simulink model "meat_1024pt_bee2_fpv3"  (Simulink 6.2)
settings: Solver=ode45  StartTime=0.0  StopTime=60000  RelTol=1e-3
undefined symbols (not defined in the file): BEE2_usr, bit_rev, pfb_coeff_gen_calc
libraries: xbsIndex_r3 x1085, casper_library x94, xps_library x27
(part 3 of 8)

== system meat_1024pt_bee2_fpv3/vacc2 ==
  note: The slice selects the upper bits of the
      | counter which represent the vector number.
  note: Acc Len is the total number of vectors accumulated minus one
      | Thus acc_len = 0 causes no accumulation, the data is passed through
  note: Valid goes high when dout
      | represents a valid accumulation
  note: ValidDelay should be equal to
      | Add Latency + Mux Latency to align the valid pulse with the output data.
  note: We want to generate a sync pulse that
      | will reset the counter right when the low bits
      | would roll over from veclen-1 to 0 so we need
      | to compare to veclen-2 to take into account
      | the latency in the comparator
  sync : Inport  Port=1  LatchInput=off
  din : Inport  Port=2  LatchInput=off
  acc_len : Inport  Port=3  LatchInput=off
  AND : xbsIndex_r3/Logical  logical_function=AND  inputs=2  precision=Full  arith_type=Unsigned  n_bits=8  bin_pt=2  align_bp=on  latency=0  explicit_period=off  period=1  en=off  dbl_ovrd=off  show_param=off
      settings: xl_area=[0, 0, 0, 0, 0, 0, 0]
  AccEnCompare : xbsIndex_r3/Relational  mode=a!=b  latency=1  explicit_period=off  period=1  en=off  dbl_ovrd=off  show_param=off
      settings: xl_area=[0, 0, 0, 0, 0, 0, 0]
  Counter : xbsIndex_r3/Counter  cnt_type=Free Running  n_bits=20  bin_pt=0  arith_type=Unsigned  start_count=0  cnt_to=Inf  cnt_by_val=1  operation=Up  explicit_period=on  period=1  load_pin=off  rst=on  en=off  dbl_ovrd=off  show_param=off  use_rpm=on  gen_core=off
      settings: xl_area=[0, 0, 0, 0, 0, 0, 0]
  Cram : Subsystem  AncestorBlock=gavrt_library/cram  mask(cram){num_slice=2}
      mask prompts: num_slice "Number of slices"
      mask help: Concatenates inputs together after forcing binary point to zero.
      mask init:
      | cram_init(gcb, ...
      |     'num_slice', num_slice);
  DinDelay : xbsIndex_r3/Delay  latency=2  reg_retiming=on  explicit_period=off  period=1  en=off  accept_only_valid=off  init_zero=on  dbl_ovrd=off  show_param=off
      settings: xl_area=[0, 0, 0, 0, 0, 0, 0]
  OR : xbsIndex_r3/Logical  logical_function=OR  inputs=2  precision=Full  arith_type=Unsigned  n_bits=8  bin_pt=2  align_bp=on  latency=0  explicit_period=off  period=1  en=off  dbl_ovrd=off  show_param=off
      settings: xl_area=[0, 0, 0, 0, 0, 0, 0]
  Slice : xbsIndex_r3/Slice  mode=Upper Bit Location + Width  nbits=10  bit1=0  base1=MSB of Input  bit0=0  base0=LSB of Input  boolean_output=off  explicit_period=off  period=1  dbl_ovrd=off
  SliceLow : xbsIndex_r3/Slice  mode=Lower Bit Location + Width  nbits=10  bit1=0  base1=MSB of Input  bit0=0  base0=LSB of Input  boolean_output=off  explicit_period=off  period=1  dbl_ovrd=off
  SyncCompare : xbsIndex_r3/Relational  mode=a=b  latency=1  explicit_period=off  period=1  en=off  dbl_ovrd=off  show_param=off
      settings: xl_area=[0, 0, 0, 0, 0, 0, 0]
  SyncConst : xbsIndex_r3/Constant  const=1022  equ=P=C  arith_type=Unsigned  n_bits=10  bin_pt=0  opselect=C  inp2=PCIN>>17  opr=+  inp1=P  carry=CIN  iostate=0  explicit_period=on  period=1  dbl_ovrd=off
  SyncDelay : xbsIndex_r3/Delay  latency=0  reg_retiming=off  explicit_period=off  period=1  en=off  accept_only_valid=off  init_zero=on  dbl_ovrd=off  show_param=off
      settings: xl_area=[0, 0, 0, 0, 0, 0, 0]
  Uncram : Subsystem  AncestorBlock=gavrt_library/uncram  mask(uncram){num_slice=2, slice_width=48, bin_pt=46, arith_type=0}
      mask prompts: num_slice "Number of slices"; slice_width "Slice Width"; bin_pt "Output Binary Point"; arith_type "Output Arithmetic Type (0=Unsigned, 1=Signed, 2=Boolean)"
      mask help: Takes a concatenated input and slices it up into even pieces and reinterprets them as signed fixed point numbers with a given binary point.
      mask init:
      | uncram_init(gcb, ...
      |     'num_slice', num_slice, ...
      |     'slice_width', slice_width, ...
      |     'bin_pt', bin_pt, ...
      |     'arith_type', arith_type);
      settings: AttributesFormatString=UFix_48_46
  ValidCompare : xbsIndex_r3/Relational  mode=a=b  latency=1  explicit_period=off  period=1  en=off  dbl_ovrd=off  show_param=off
      settings: xl_area=[0, 0, 0, 0, 0, 0, 0]
  ValidDelay : xbsIndex_r3/Delay  latency=3  reg_retiming=off  explicit_period=off  period=1  en=off  accept_only_valid=off  init_zero=on  dbl_ovrd=off  show_param=off
      settings: xl_area=[0, 0, 0, 0, 0, 0, 0]
  Zero : xbsIndex_r3/Constant  const=0  equ=P=C  arith_type=Unsigned  n_bits=8  bin_pt=0  opselect=C  inp2=PCIN>>17  opr=+  inp1=P  carry=CIN  iostate=0  explicit_period=on  period=1  dbl_ovrd=off
  vacc_core1 : Subsystem  AncestorBlock=gavrt_library/vacc_core  mask(vacc_core){veclen=1024, arith_type=0, out_bit_width=64, out_bin_pt=46, add_latency=2, bram_latency=2, mux_latency=1}
      mask prompts: veclen "Vector Length"; arith_type "Arithmetic Type (0=Unsigned, 1=Signed)"; out_bit_width "Output Bit Width"; out_bin_pt "Output Binary Point"; add_latency "Add Latency"; bram_latency "BRAM Latency"; mux_latency "Mux Latency"
      mask help:
      | Currently only Signed arithmetic supported
      | acc_en = 0 --> Load a vector (start a new accumulation)
      | acc_en = 1 --> Accumulate
      mask init: same as meat_1024pt_bee2_fpv3/vacc/vacc_core1
  vacc_core2 : Subsystem  AncestorBlock=gavrt_library/vacc_core  mask(vacc_core){veclen=1024, arith_type=0, out_bit_width=64, out_bin_pt=46, add_latency=2, bram_latency=2, mux_latency=1}
      mask prompts: veclen "Vector Length"; arith_type "Arithmetic Type (0=Unsigned, 1=Signed)"; out_bit_width "Output Bit Width"; out_bin_pt "Output Binary Point"; add_latency "Add Latency"; bram_latency "BRAM Latency"; mux_latency "Mux Latency"
      mask help:
      | Currently only Signed arithmetic supported
      | acc_en = 0 --> Load a vector (start a new accumulation)
      | acc_en = 1 --> Accumulate
      mask init: same as meat_1024pt_bee2_fpv3/vacc/vacc_core1
  valid : Outport
  dout : Outport  Port=2
  wires:
  sync/1 -> SyncDelay/1
  SyncDelay/1 -> OR/1
  [valid] -> AND/1
  AND/1 -> OR/2
  OR/1 -> Counter/1
  Counter/1 -> [count], Slice/1
  [count] -> SliceLow/1
  SliceLow/1 -> SyncCompare/1
  SyncConst/1 -> SyncCompare/2
  SyncCompare/1 -> AND/2
  ValidCompare/1 -> [valid], ValidDelay/1
  acc_len/1 -> ValidCompare/1
  Slice/1 -> ValidCompare/2, AccEnCompare/1
  Zero/1 -> AccEnCompare/2
  ValidDelay/1 -> valid/1
  din/1 -> DinDelay/1
  DinDelay/1 -> Uncram/1(In)
  Cram/1(Out) -> dout/1
  Uncram/1(Out1) -> vacc_core1/1(din)
  AccEnCompare/1 -> vacc_core1/2(acc_en), vacc_core2/2(acc_en)
  vacc_core1/1(dout) -> Cram/1(In1)
  Uncram/2(Out2) -> vacc_core2/1(din)
  vacc_core2/1(dout) -> Cram/2(In2)

== system meat_1024pt_bee2_fpv3/StokesDetector/XMultiply_f0 ==
  Pol1 : Inport  Port=1  LatchInput=off
  Pol2 : Inport  Port=2  LatchInput=off
  add : xbsIndex_r3/AddSub  mode=Addition  precision=User Defined  arith_type="Signed  (2's comp)"  n_bits=32  bin_pt=31  quantization="Round  (unbiased: +/- Inf)"  overflow=Wrap  latency=2  explicit_period=off  period=1  use_carryin=off  use_carryout=off  en=off  dbl_ovrd=off  show_param=off  use_core=on  pipeline=off  use_rpm=on  gen_core=off
      settings: xl_area=[0, 0, 0, 0, 0, 0, 0]
  c_to_ri : casper_library/Misc/c_to_ri  n_bits=18  bin_pt=17
      settings: AttributesFormatString=18_17 r/i
  c_to_ri1 : casper_library/Misc/c_to_ri  n_bits=18  bin_pt=17
      settings: AttributesFormatString=18_17 r/i
  mult{1..4} (4 alike) : xbsIndex_r3/Mult  precision=Full  arith_type="Signed  (2's comp)"  n_bits=8  bin_pt=2  quantization=Truncate  overflow=Wrap  latency=3  explicit_period=off  period=1  en=off  dbl_ovrd=off  show_param=on  mult_type=Parallel  oversample=2  use_embedded=on  pipeline=on  use_rpm=on  placement_style=Rectangular Shape  gen_core=off
      settings: xl_area=[0, 0, 0, 0, 0, 0, 0]
  sub : xbsIndex_r3/AddSub  mode=Subtraction  precision=User Defined  arith_type="Signed  (2's comp)"  n_bits=32  bin_pt=31  quantization="Round  (unbiased: +/- Inf)"  overflow=Wrap  latency=2  explicit_period=off  period=1  use_carryin=off  use_carryout=off  en=off  dbl_ovrd=off  show_param=off  use_core=on  pipeline=off  use_rpm=on  gen_core=off
      settings: xl_area=[0, 0, 0, 0, 0, 0, 0]
  X Real : Outport
  X Imag : Outport  Port=2
  wires:
  c_to_ri/1 -> mult1/1, mult2/1
  c_to_ri1/1 -> mult1/2, mult3/2
  c_to_ri/2 -> mult3/1, mult4/1
  c_to_ri1/2 -> mult2/2, mult4/2
  mult4/1 -> add/1
  mult1/1 -> add/2
  mult2/1 -> sub/1
  mult3/1 -> sub/2
  Pol1/1 -> c_to_ri/1
  Pol2/1 -> c_to_ri1/1
  add/1 -> X Real/1
  sub/1 -> X Imag/1

== system meat_1024pt_bee2_fpv3/StokesDetector/pol1_power0 ==
  note: Power - Unsigned Output
  c : Inport  Port=1  LatchInput=off
  c_to_ri : casper_library/Misc/c_to_ri  n_bits=18  bin_pt=17
      settings: AttributesFormatString=18_17 r/i
  imag_square : xbsIndex_r3/Mult  precision=Full  arith_type="Signed  (2's comp)"  n_bits=18  bin_pt=17  quantization=Truncate  overflow=Wrap  latency=3  explicit_period=off  period=1  en=off  dbl_ovrd=off  show_param=on  mult_type=Parallel  oversample=2  use_embedded=on  pipeline=on  use_rpm=on  placement_style=Rectangular Shape  gen_core=off
      settings: xl_area=[0, 0, 0, 0, 0, 0, 0]
  power_adder : xbsIndex_r3/AddSub  mode=Addition  precision=User Defined  arith_type=Unsigned  n_bits=32  bin_pt=31  quantization="Round  (unbiased: +/- Inf)"  overflow=Wrap  latency=2  explicit_period=off  period=1  use_carryin=off  use_carryout=off  en=off  dbl_ovrd=off  show_param=off  use_core=on  pipeline=off  use_rpm=on  gen_core=off
      settings: xl_area=[0, 0, 0, 0, 0, 0, 0]
  real_square : xbsIndex_r3/Mult  precision=Full  arith_type="Signed  (2's comp)"  n_bits=18  bin_pt=17  quantization=Truncate  overflow=Wrap  latency=3  explicit_period=off  period=1  en=off  dbl_ovrd=off  show_param=on  mult_type=Parallel  oversample=2  use_embedded=on  pipeline=on  use_rpm=on  placement_style=Rectangular Shape  gen_core=off
      settings: xl_area=[0, 0, 0, 0, 0, 0, 0]
  power : Outport
  wires:
  imag_square/1 -> power_adder/2
  real_square/1 -> power_adder/1
  c_to_ri/1 -> real_square/1, real_square/2
  c_to_ri/2 -> imag_square/2, imag_square/1
  c/1 -> c_to_ri/1
  power_adder/1 -> power/1

== system meat_1024pt_bee2_fpv3/StokesDetector/pol2_power0 ==
  note: Power - Unsigned Output
  c : Inport  Port=1  LatchInput=off
  c_to_ri : casper_library/Misc/c_to_ri  n_bits=18  bin_pt=17
      settings: AttributesFormatString=18_17 r/i
  imag_square : xbsIndex_r3/Mult  precision=Full  arith_type="Signed  (2's comp)"  n_bits=18  bin_pt=17  quantization=Truncate  overflow=Wrap  latency=3  explicit_period=off  period=1  en=off  dbl_ovrd=off  show_param=on  mult_type=Parallel  oversample=2  use_embedded=on  pipeline=on  use_rpm=on  placement_style=Rectangular Shape  gen_core=off
      settings: xl_area=[0, 0, 0, 0, 0, 0, 0]
  power_adder : xbsIndex_r3/AddSub  mode=Addition  precision=User Defined  arith_type=Unsigned  n_bits=32  bin_pt=31  quantization="Round  (unbiased: +/- Inf)"  overflow=Wrap  latency=2  explicit_period=off  period=1  use_carryin=off  use_carryout=off  en=off  dbl_ovrd=off  show_param=off  use_core=on  pipeline=off  use_rpm=on  gen_core=off
      settings: xl_area=[0, 0, 0, 0, 0, 0, 0]
  real_square : xbsIndex_r3/Mult  precision=Full  arith_type="Signed  (2's comp)"  n_bits=18  bin_pt=17  quantization=Truncate  overflow=Wrap  latency=3  explicit_period=off  period=1  en=off  dbl_ovrd=off  show_param=on  mult_type=Parallel  oversample=2  use_embedded=on  pipeline=on  use_rpm=on  placement_style=Rectangular Shape  gen_core=off
      settings: xl_area=[0, 0, 0, 0, 0, 0, 0]
  power : Outport
  wires:
  power_adder/1 -> power/1
  c/1 -> c_to_ri/1
  c_to_ri/2 -> imag_square/1, imag_square/2
  c_to_ri/1 -> real_square/2, real_square/1
  real_square/1 -> power_adder/1
  imag_square/1 -> power_adder/2

== system meat_1024pt_bee2_fpv3/fft/fft_biplex0 ==
  pol1 : Inport  Port=1  LatchInput=off
  pol2 : Inport  Port=2  LatchInput=off
  sync : Inport  Port=3  LatchInput=off
  shift : Inport  Port=4  LatchInput=off
  biplex_core : Subsystem  AncestorBlock=casper_library/FFTs/biplex_core  mask(biplex_core){FFTSize=10, BitWidth=18, quantization=Truncate, overflow=Wrap, add_latency=3, mult_latency=4, bram_latency=3}
      mask prompts: FFTSize "Size of FFT: (2^? pnts)"; BitWidth "Bitwidth: (Max Efficiency at 18 bits)"; quantization "Quantization Behavior"; overflow "Overflow Behavior"; add_latency "Add Latency"; mult_latency "Mult Latency"; bram_latency "BRAM Latency"
      mask init:
      | biplex_core_init(gcb,...
      |     'FFTSize', FFTSize,...
      |     'BitWidth', BitWidth,...
      |     'quantization', quantization,...
      |     'overflow', overflow,...
      |     'add_latency', add_latency,...
      |     'mult_latency', mult_latency,...
      |     'bram_latency', bram_latency);
      settings: AttributesFormatString=FFTSize=10
      mask StyleString: edit,edit,popup(Truncate|Round  (unbiased: +/- Inf)|Round  (unbiased: Even Values)),popup(Wrap|Saturate|Error),edit,edit,edit
  biplex_cplx_unscrambler : Subsystem  mask{FFTSize=10, bram_latency=3}
      mask prompts: FFTSize "Size of FFT: (2^? pnts)"; bram_latency "BRAM Latency"
      mask init:
      | blk = gcb;
      | map = bit_reverse(0:2^(FFTSize-1)-1, FFTSize-1);
      | set_param([blk,'/reorder'],'map',mat2str([map,map+2^(FFTSize-1)]));
      | set_param([blk,'/reorder'],'bram_latency', num2str(bram_latency));
      | set_param([blk,'/reorder1'],'map',mat2str([map+2^(FFTSize-1),map]));
      | set_param([blk,'/reorder1'],'bram_latency', num2str(bram_latency));
  pol1_out : Outport
  pol2_out : Outport  Port=2
  of : Outport  Port=3
  sync_out : Outport  Port=4
  wires:
  biplex_cplx_unscrambler/3(sync_out) -> sync_out/1
  biplex_cplx_unscrambler/2(pol2) -> pol2_out/1
  biplex_core/4(sync_out) -> biplex_cplx_unscrambler/3(sync)
  biplex_core/2(out2) -> biplex_cplx_unscrambler/2(odd)
  biplex_core/1(out1) -> biplex_cplx_unscrambler/1(even)
  pol1/1 -> biplex_core/1(pol1)
  pol2/1 -> biplex_core/2(pol2)
  sync/1 -> biplex_core/3(sync)
  shift/1 -> biplex_core/4(shift)
  biplex_cplx_unscrambler/1(pol1) -> pol1_out/1
  biplex_core/3(of) -> of/1

== system meat_1024pt_bee2_fpv3/pfb_fir/pol1_in1_first_tap ==
  din : Inport  Port=1  LatchInput=off
  sync : Inport  Port=2  LatchInput=off
  Mult : xbsIndex_r3/Mult  precision=Full  arith_type="Signed  (2's comp)"  n_bits=8  bin_pt=2  quantization=Truncate  overflow=Wrap  latency=mult_latency  explicit_period=off  period=1  en=off  dbl_ovrd=off  show_param=on  mult_type=Parallel  oversample=2  use_embedded=on  pipeline=on  use_rpm=on  placement_style=Rectangular Shape  gen_core=off
      settings: xl_area=[0, 0, 0, 0, 0, 0, 0]
  Mult1 : xbsIndex_r3/Mult  precision=Full  arith_type="Signed  (2's comp)"  n_bits=8  bin_pt=2  quantization=Truncate  overflow=Wrap  latency=mult_latency  explicit_period=off  period=1  en=off  dbl_ovrd=off  show_param=on  mult_type=Parallel  oversample=2  use_embedded=on  pipeline=on  use_rpm=on  placement_style=Rectangular Shape  gen_core=off
      settings: xl_area=[0, 0, 0, 0, 0, 0, 0]
  Reinterpret : xbsIndex_r3/Reinterpret  force_arith_type=on  arith_type="Signed  (2's comp)"  force_bin_pt=on  bin_pt=CoeffBitWidth - 1  force_valid=on
  Slice : xbsIndex_r3/Slice  mode=Lower Bit Location + Width  nbits=CoeffBitWidth  bit1=0  base1=MSB of Input  bit0=0  base0=LSB of Input  boolean_output=off  explicit_period=off  period=1  dbl_ovrd=off
  Slice1 : xbsIndex_r3/Slice  mode=Two Bit Locations  nbits=CoeffBitWidth * (TotalTaps - 1)  bit1=0  base1=MSB of Input  bit0=CoeffBitWidth  base0=LSB of Input  boolean_output=off  explicit_period=off  period=1  dbl_ovrd=off
  c_to_ri : casper_library/Misc/c_to_ri  n_bits=BitWidthIn  bin_pt=BitWidthIn-1
      settings: AttributesFormatString=8_7 r/i
  delay : Subsystem  BlockChoice=delay_bram
      link override delay_bram: DelayLen=2^(PFBSize-n_inputs)  bram_latency=bram_latency
      link override delay_bram/Constant2: equ=P=C
      settings: AttributesFormatString=%<BlockChoice>  TemplateBlock=casper_library/Delays/delay  MemberBlocks=delay_bram,delay_slr
  pfb_coeff_gen : Subsystem  AncestorBlock=casper_library/PFBs/pfb_coeff_gen  mask(pfb_coeff_gen){PFBSize=10, CoeffBitWidth=8, TotalTaps=4, CoeffDistMem=1, WindowType=hamming, bram_latency=3, n_inputs=0, nput=0, fwidth=1}
      mask prompts: PFBSize "Size of PFB: (2^? pnts)"; CoeffBitWidth "Bitwidth of Coefficients:"; TotalTaps "Total Number of Taps:"; CoeffDistMem "Implement Coeff Gen in Distributed Memory"; WindowType "Windowing Function:"; bram_latency "BRAM Latency"; n_inputs "Number of Simultaneous Inputs: (2^?)"; nput "This is input number:"; fwidth "Bin Width (normal=1)"
      mask init:
      | pfb_coeff_gen_init(gcb, ...
      |     'PFBSize', PFBSize, ...
      |     'CoeffBitWidth', CoeffBitWidth, ...
      |     'TotalTaps', TotalTaps, ...
      |     'CoeffDistMem', CoeffDistMem, ...
      |     'WindowType', WindowType, ...
      |     'bram_latency', bram_latency, ...
      |     'n_inputs', n_inputs, ...
      |     'nput', nput, ...
      |     'fwidth', fwidth);
      settings: AttributesFormatString=PFBSize=10, n_inputs=0, taps=4
  ri_to_c : Subsystem
  sync_delay : casper_library/Delays/sync_delay  DelayLen=2^(PFBSize-n_inputs)
      link override Constant: equ=P=C
      link override Constant1: equ=P=C
      link override Constant2: equ=P=C
      link override Constant3: equ=P=C
  dout : Outport
  sync_out : Outport  Port=2
  coeff_out : Outport  Port=3
  taps_out : Outport  Port=4
  wires:
  ri_to_c/1(c) -> taps_out/1
  Mult/1 -> ri_to_c/2(im)
  Mult1/1 -> ri_to_c/1(re)
  c_to_ri/2 -> Mult/1
  c_to_ri/1 -> Mult1/1
  pfb_coeff_gen/3(coeff) -> Slice1/1, Slice/1
  pfb_coeff_gen/2(sync_out) -> sync_delay/1
  sync/1 -> pfb_coeff_gen/2(sync)
  pfb_coeff_gen/1(dout) -> delay/1(In1), c_to_ri/1
  din/1 -> pfb_coeff_gen/1(din)
  delay/1(Out1) -> dout/1
  sync_delay/1 -> sync_out/1
  Slice1/1 -> coeff_out/1
  Slice/1 -> Reinterpret/1
  Reinterpret/1 -> Mult1/2, Mult/2

== system meat_1024pt_bee2_fpv3/pfb_fir/pol1_in1_last_tap ==
  din : Inport  Port=1  LatchInput=off
  sync : Inport  Port=2  LatchInput=off
  coeff : Inport  Port=3  LatchInput=off
  taps : Inport  Port=4  LatchInput=off
  Concat : xbsIndex_r3/Concat  num_inputs=2  explicit_period=off  period=1  dbl_ovrd=off
  Delay : xbsIndex_r3/Delay  latency=mult_latency  reg_retiming=off  explicit_period=off  period=1  en=off  accept_only_valid=off  init_zero=on  dbl_ovrd=off  show_param=off
      settings: xl_area=[0, 0, 0, 0, 0, 0, 0]
  Mult : xbsIndex_r3/Mult  precision=Full  arith_type="Signed  (2's comp)"  n_bits=8  bin_pt=2  quantization=Truncate  overflow=Wrap  latency=mult_latency  explicit_period=off  period=1  en=off  dbl_ovrd=off  show_param=on  mult_type=Parallel  oversample=2  use_embedded=on  pipeline=on  use_rpm=on  placement_style=Rectangular Shape  gen_core=off
      settings: xl_area=[0, 0, 0, 0, 0, 0, 0]
  Mult1 : xbsIndex_r3/Mult  precision=Full  arith_type="Signed  (2's comp)"  n_bits=8  bin_pt=2  quantization=Truncate  overflow=Wrap  latency=mult_latency  explicit_period=off  period=1  en=off  dbl_ovrd=off  show_param=on  mult_type=Parallel  oversample=2  use_embedded=on  pipeline=on  use_rpm=on  placement_style=Rectangular Shape  gen_core=off
      settings: xl_area=[0, 0, 0, 0, 0, 0, 0]
  Reinterpret : xbsIndex_r3/Reinterpret  force_arith_type=on  arith_type="Signed  (2's comp)"  force_bin_pt=on  bin_pt=CoeffBitWidth - 1  force_valid=on
  c_to_ri : casper_library/Misc/c_to_ri  n_bits=BitWidthIn  bin_pt=BitWidthIn-1
      settings: AttributesFormatString=8_7 r/i
  pfb_add_tree : Subsystem  mask(pfb_add_tree){TotalTaps=4, BitWidthIn=8, BitWidthOut=18, CoeffBitWidth=8, add_latency=2, quantization=Truncate}
      mask prompts: TotalTaps "Total Number of Taps:"; BitWidthIn "Input Bitwidth:"; BitWidthOut "Output Bitwidth:"; CoeffBitWidth "Coeff Bitwidth:"; add_latency "Add Latency"; quantization "Quantization Behavior"
      mask init:
      | pfb_add_tree_init(gcb, ...
      |     'TotalTaps', TotalTaps, ...
      |     'BitWidthIn', BitWidthIn, ...
      |     'BitWidthOut', BitWidthOut, ...
      |     'CoeffBitWidth', CoeffBitWidth, ...
      |     'add_latency', add_latency, ...
      |     'quantization', quantization);
      settings: AttributesFormatString=taps=4, add_latency=2
  ri_to_c : Subsystem
  dout : Outport
  sync_out : Outport  Port=2
  wires:
  Reinterpret/1 -> Mult/2, Mult1/2
  coeff/1 -> Reinterpret/1
  Concat/1 -> pfb_add_tree/1(din)
  taps/1 -> Concat/2
  sync/1 -> Delay/1
  pfb_add_tree/1(dout) -> dout/1
  pfb_add_tree/2(sync_out) -> sync_out/1
  Delay/1 -> pfb_add_tree/2(sync)
  c_to_ri/1 -> Mult1/1
  c_to_ri/2 -> Mult/1
  din/1 -> c_to_ri/1
  Mult1/1 -> ri_to_c/1(re)
  Mult/1 -> ri_to_c/2(im)
  ri_to_c/1(c) -> Concat/1

== system meat_1024pt_bee2_fpv3/pfb_fir/pol2_in1_first_tap ==
  din : Inport  Port=1  LatchInput=off
  sync : Inport  Port=2  LatchInput=off
  Mult : xbsIndex_r3/Mult  precision=Full  arith_type="Signed  (2's comp)"  n_bits=8  bin_pt=2  quantization=Truncate  overflow=Wrap  latency=mult_latency  explicit_period=off  period=1  en=off  dbl_ovrd=off  show_param=on  mult_type=Parallel  oversample=2  use_embedded=on  pipeline=on  use_rpm=on  placement_style=Rectangular Shape  gen_core=off
      settings: xl_area=[0, 0, 0, 0, 0, 0, 0]
  Mult1 : xbsIndex_r3/Mult  precision=Full  arith_type="Signed  (2's comp)"  n_bits=8  bin_pt=2  quantization=Truncate  overflow=Wrap  latency=mult_latency  explicit_period=off  period=1  en=off  dbl_ovrd=off  show_param=on  mult_type=Parallel  oversample=2  use_embedded=on  pipeline=on  use_rpm=on  placement_style=Rectangular Shape  gen_core=off
      settings: xl_area=[0, 0, 0, 0, 0, 0, 0]
  Reinterpret : xbsIndex_r3/Reinterpret  force_arith_type=on  arith_type="Signed  (2's comp)"  force_bin_pt=on  bin_pt=CoeffBitWidth - 1  force_valid=on
  Slice : xbsIndex_r3/Slice  mode=Lower Bit Location + Width  nbits=CoeffBitWidth  bit1=0  base1=MSB of Input  bit0=0  base0=LSB of Input  boolean_output=off  explicit_period=off  period=1  dbl_ovrd=off
  Slice1 : xbsIndex_r3/Slice  mode=Two Bit Locations  nbits=CoeffBitWidth * (TotalTaps - 1)  bit1=0  base1=MSB of Input  bit0=CoeffBitWidth  base0=LSB of Input  boolean_output=off  explicit_period=off  period=1  dbl_ovrd=off
  c_to_ri : casper_library/Misc/c_to_ri  n_bits=BitWidthIn  bin_pt=BitWidthIn-1
      settings: AttributesFormatString=8_7 r/i
  delay : Subsystem  BlockChoice=delay_bram
      link override delay_bram: DelayLen=2^(PFBSize-n_inputs)  bram_latency=bram_latency
      link override delay_bram/Constant2: equ=P=C
      settings: AttributesFormatString=%<BlockChoice>  TemplateBlock=casper_library/Delays/delay  MemberBlocks=delay_bram,delay_slr
  pfb_coeff_gen : Subsystem  AncestorBlock=casper_library/PFBs/pfb_coeff_gen  mask(pfb_coeff_gen){PFBSize=10, CoeffBitWidth=8, TotalTaps=4, CoeffDistMem=1, WindowType=hamming, bram_latency=3, n_inputs=0, nput=0, fwidth=1}
      mask prompts: PFBSize "Size of PFB: (2^? pnts)"; CoeffBitWidth "Bitwidth of Coefficients:"; TotalTaps "Total Number of Taps:"; CoeffDistMem "Implement Coeff Gen in Distributed Memory"; WindowType "Windowing Function:"; bram_latency "BRAM Latency"; n_inputs "Number of Simultaneous Inputs: (2^?)"; nput "This is input number:"; fwidth "Bin Width (normal=1)"
      mask init: same as meat_1024pt_bee2_fpv3/pfb_fir/pol1_in1_first_tap/pfb_coeff_gen
      settings: AttributesFormatString=PFBSize=10, n_inputs=0, taps=4
  ri_to_c : Subsystem
  sync_delay : casper_library/Delays/sync_delay  DelayLen=2^(PFBSize-n_inputs)
      link override Constant: equ=P=C
      link override Constant1: equ=P=C
      link override Constant2: equ=P=C
      link override Constant3: equ=P=C
  dout : Outport
  sync_out : Outport  Port=2
  coeff_out : Outport  Port=3
  taps_out : Outport  Port=4
  wires:
  ri_to_c/1(c) -> taps_out/1
  Mult/1 -> ri_to_c/2(im)
  Mult1/1 -> ri_to_c/1(re)
  c_to_ri/2 -> Mult/1
  c_to_ri/1 -> Mult1/1
  pfb_coeff_gen/3(coeff) -> Slice1/1, Slice/1
  pfb_coeff_gen/2(sync_out) -> sync_delay/1
  sync/1 -> pfb_coeff_gen/2(sync)
  pfb_coeff_gen/1(dout) -> delay/1(In1), c_to_ri/1
  din/1 -> pfb_coeff_gen/1(din)
  delay/1(Out1) -> dout/1
  sync_delay/1 -> sync_out/1
  Slice1/1 -> coeff_out/1
  Slice/1 -> Reinterpret/1
  Reinterpret/1 -> Mult1/2, Mult/2

== system meat_1024pt_bee2_fpv3/pfb_fir/pol2_in1_last_tap ==
  din : Inport  Port=1  LatchInput=off
  sync : Inport  Port=2  LatchInput=off
  coeff : Inport  Port=3  LatchInput=off
  taps : Inport  Port=4  LatchInput=off
  Concat : xbsIndex_r3/Concat  num_inputs=2  explicit_period=off  period=1  dbl_ovrd=off
  Delay : xbsIndex_r3/Delay  latency=mult_latency  reg_retiming=off  explicit_period=off  period=1  en=off  accept_only_valid=off  init_zero=on  dbl_ovrd=off  show_param=off
      settings: xl_area=[0, 0, 0, 0, 0, 0, 0]
  Mult : xbsIndex_r3/Mult  precision=Full  arith_type="Signed  (2's comp)"  n_bits=8  bin_pt=2  quantization=Truncate  overflow=Wrap  latency=mult_latency  explicit_period=off  period=1  en=off  dbl_ovrd=off  show_param=on  mult_type=Parallel  oversample=2  use_embedded=on  pipeline=on  use_rpm=on  placement_style=Rectangular Shape  gen_core=off
      settings: xl_area=[0, 0, 0, 0, 0, 0, 0]
  Mult1 : xbsIndex_r3/Mult  precision=Full  arith_type="Signed  (2's comp)"  n_bits=8  bin_pt=2  quantization=Truncate  overflow=Wrap  latency=mult_latency  explicit_period=off  period=1  en=off  dbl_ovrd=off  show_param=on  mult_type=Parallel  oversample=2  use_embedded=on  pipeline=on  use_rpm=on  placement_style=Rectangular Shape  gen_core=off
      settings: xl_area=[0, 0, 0, 0, 0, 0, 0]
  Reinterpret : xbsIndex_r3/Reinterpret  force_arith_type=on  arith_type="Signed  (2's comp)"  force_bin_pt=on  bin_pt=CoeffBitWidth - 1  force_valid=on
  c_to_ri : casper_library/Misc/c_to_ri  n_bits=BitWidthIn  bin_pt=BitWidthIn-1
      settings: AttributesFormatString=8_7 r/i
  pfb_add_tree : Subsystem  mask(pfb_add_tree){TotalTaps=4, BitWidthIn=8, BitWidthOut=18, CoeffBitWidth=8, add_latency=2, quantization=Truncate}
      mask prompts: TotalTaps "Total Number of Taps:"; BitWidthIn "Input Bitwidth:"; BitWidthOut "Output Bitwidth:"; CoeffBitWidth "Coeff Bitwidth:"; add_latency "Add Latency"; quantization "Quantization Behavior"
      mask init: same as meat_1024pt_bee2_fpv3/pfb_fir/pol1_in1_last_tap/pfb_add_tree
      settings: AttributesFormatString=taps=4, add_latency=2
  ri_to_c : Subsystem
  dout : Outport
  sync_out : Outport  Port=2
  wires:
  Reinterpret/1 -> Mult/2, Mult1/2
  coeff/1 -> Reinterpret/1
  Concat/1 -> pfb_add_tree/1(din)
  taps/1 -> Concat/2
  sync/1 -> Delay/1
  pfb_add_tree/1(dout) -> dout/1
  pfb_add_tree/2(sync_out) -> sync_out/1
  Delay/1 -> pfb_add_tree/2(sync)
  c_to_ri/1 -> Mult1/1
  c_to_ri/2 -> Mult/1
  din/1 -> c_to_ri/1
  Mult1/1 -> ri_to_c/1(re)
  Mult/1 -> ri_to_c/2(im)
  ri_to_c/1(c) -> Concat/1

== system meat_1024pt_bee2_fpv3/vacc/Cram ==
  In1 : Inport  Port=1  LatchInput=off
  In2 : Inport  Port=2  LatchInput=off
  Concat : xbsIndex_r3/Concat  num_inputs=2  explicit_period=off  period=1  dbl_ovrd=off
  Reinterp1 : xbsIndex_r3/Reinterpret  force_arith_type=on  arith_type=Unsigned  force_bin_pt=on  bin_pt=0  force_valid=on
  Reinterp2 : xbsIndex_r3/Reinterpret  force_arith_type=on  arith_type=Unsigned  force_bin_pt=on  bin_pt=0  force_valid=on
  Out : Outport
  wires:
  Concat/1 -> Out/1
  In1/1 -> Reinterp1/1
  Reinterp1/1 -> Concat/1
  In2/1 -> Reinterp2/1
  Reinterp2/1 -> Concat/2

== system meat_1024pt_bee2_fpv3/vacc/Uncram ==
  In : Inport  Port=1  LatchInput=off
  Reinterp1 : xbsIndex_r3/Reinterpret  force_arith_type=on  arith_type="Signed  (2's comp)"  force_bin_pt=on  bin_pt=31  force_valid=on
  Reinterp2 : xbsIndex_r3/Reinterpret  force_arith_type=on  arith_type="Signed  (2's comp)"  force_bin_pt=on  bin_pt=31  force_valid=on
  Slice1 : xbsIndex_r3/Slice  mode=Upper Bit Location + Width  nbits=32  bit1=0  base1=MSB of Input  bit0=0  base0=LSB of Input  boolean_output=off  explicit_period=off  period=1  dbl_ovrd=off
  Slice2 : xbsIndex_r3/Slice  mode=Upper Bit Location + Width  nbits=32  bit1=-32  base1=MSB of Input  bit0=0  base0=LSB of Input  boolean_output=off  explicit_period=off  period=1  dbl_ovrd=off
  Out1 : Outport
  Out2 : Outport  Port=2
  wires:
  In/1 -> Slice1/1, Slice2/1
  Slice1/1 -> Reinterp1/1
  Reinterp1/1 -> Out1/1
  Slice2/1 -> Reinterp2/1
  Reinterp2/1 -> Out2/1

== system meat_1024pt_bee2_fpv3/vacc/vacc_core1 ==
  note: This BRAM and counter is exactly what is inside the green
      | Delay BRAM block. The functionality was extracted to avoid
      | library issues.
  din : Inport  Port=1  LatchInput=off
  acc_en : Inport  Port=2  LatchInput=off
  Adder : xbsIndex_r3/AddSub  mode=Addition  precision=User Defined  arith_type="Signed  (2's comp)"  n_bits=48  bin_pt=31  quantization=Truncate  overflow=Wrap  latency=2  explicit_period=on  period=1  use_carryin=off  use_carryout=off  en=off  dbl_ovrd=off  show_param=on  use_core=on  pipeline=on  use_rpm=on  gen_core=off
      settings: xl_area=[0, 0, 0, 0, 0, 0, 0]
  BRAM : xbsIndex_r3/Single Port RAM  depth=1024  initVector=0  write_mode=Read Before Write  latency=2  init_zero=on  explicit_period=off  period=1  rst=off  init_reg=0  en=off  dbl_ovrd=off  show_param=off  distributed_mem=off  use_rpm=off  gen_core=off
      settings: xl_area=[0, 0, 0, 0, 0, 0, 0]
  Constant : xbsIndex_r3/Constant  const=0  equ=P=C  arith_type=Unsigned  n_bits=1  bin_pt=0  opselect=C  inp2=PCIN>>17  opr=+  inp1=P  carry=CIN  iostate=0  explicit_period=off  period=1  dbl_ovrd=off
  Constant2 : xbsIndex_r3/Constant  const=1  equ=P=C  arith_type=Boolean  n_bits=1  bin_pt=0  opselect=C  inp2=PCIN>>17  opr=+  inp1=P  carry=CIN  iostate=0  explicit_period=on  period=1  dbl_ovrd=off
  Counter : xbsIndex_r3/Counter  cnt_type=Count Limited  n_bits=10  bin_pt=0  arith_type=Unsigned  start_count=0  cnt_to=1018  cnt_by_val=1  operation=Up  explicit_period=off  period=1  load_pin=off  rst=off  en=off  dbl_ovrd=off  show_param=off  use_rpm=off  gen_core=on
      settings: xl_area=[0, 0, 0, 0, 0, 0, 0]
  Mux : xbsIndex_r3/Mux  inputs=2  precision=Full  arith_type="Signed  (2's comp)"  n_bits=8  bin_pt=2  quantization=Truncate  overflow=Wrap  latency=1  explicit_period=off  period=1  en=off  dbl_ovrd=off  show_param=on  mux_type=off  use_rpm=on  gen_core=off
      settings: xl_area=[0, 0, 0, 0, 0, 0, 0]
  dout : Outport
  wires:
  acc_en/1 -> Mux/1
  Constant/1 -> Mux/2
  BRAM/1 -> Mux/3
  din/1 -> Adder/1
  Mux/1 -> Adder/2
  Adder/1 -> dout/1, BRAM/2
  Counter/1 -> BRAM/1
  Constant2/1 -> BRAM/3

== system meat_1024pt_bee2_fpv3/vacc/vacc_core2 ==
  note: This BRAM and counter is exactly what is inside the green
      | Delay BRAM block. The functionality was extracted to avoid
      | library issues.
  din : Inport  Port=1  LatchInput=off
  acc_en : Inport  Port=2  LatchInput=off
  Adder : xbsIndex_r3/AddSub  mode=Addition  precision=User Defined  arith_type="Signed  (2's comp)"  n_bits=48  bin_pt=31  quantization=Truncate  overflow=Wrap  latency=2  explicit_period=on  period=1  use_carryin=off  use_carryout=off  en=off  dbl_ovrd=off  show_param=on  use_core=on  pipeline=on  use_rpm=on  gen_core=off
      settings: xl_area=[0, 0, 0, 0, 0, 0, 0]
  BRAM : xbsIndex_r3/Single Port RAM  depth=1024  initVector=0  write_mode=Read Before Write  latency=2  init_zero=on  explicit_period=off  period=1  rst=off  init_reg=0  en=off  dbl_ovrd=off  show_param=off  distributed_mem=off  use_rpm=off  gen_core=off
      settings: xl_area=[0, 0, 0, 0, 0, 0, 0]
  Constant : xbsIndex_r3/Constant  const=0  equ=P=C  arith_type=Unsigned  n_bits=1  bin_pt=0  opselect=C  inp2=PCIN>>17  opr=+  inp1=P  carry=CIN  iostate=0  explicit_period=off  period=1  dbl_ovrd=off
  Constant2 : xbsIndex_r3/Constant  const=1  equ=P=C  arith_type=Boolean  n_bits=1  bin_pt=0  opselect=C  inp2=PCIN>>17  opr=+  inp1=P  carry=CIN  iostate=0  explicit_period=on  period=1  dbl_ovrd=off
  Counter : xbsIndex_r3/Counter  cnt_type=Count Limited  n_bits=10  bin_pt=0  arith_type=Unsigned  start_count=0  cnt_to=1018  cnt_by_val=1  operation=Up  explicit_period=off  period=1  load_pin=off  rst=off  en=off  dbl_ovrd=off  show_param=off  use_rpm=off  gen_core=on
      settings: xl_area=[0, 0, 0, 0, 0, 0, 0]
  Mux : xbsIndex_r3/Mux  inputs=2  precision=Full  arith_type="Signed  (2's comp)"  n_bits=8  bin_pt=2  quantization=Truncate  overflow=Wrap  latency=1  explicit_period=off  period=1  en=off  dbl_ovrd=off  show_param=on  mux_type=off  use_rpm=on  gen_core=off
      settings: xl_area=[0, 0, 0, 0, 0, 0, 0]
  dout : Outport
  wires:
  acc_en/1 -> Mux/1
  Constant/1 -> Mux/2
  BRAM/1 -> Mux/3
  din/1 -> Adder/1
  Mux/1 -> Adder/2
  Adder/1 -> dout/1, BRAM/2
  Counter/1 -> BRAM/1
  Constant2/1 -> BRAM/3

== system meat_1024pt_bee2_fpv3/vacc1/Cram ==
  In1 : Inport  Port=1  LatchInput=off
  In2 : Inport  Port=2  LatchInput=off
  Concat : xbsIndex_r3/Concat  num_inputs=2  explicit_period=off  period=1  dbl_ovrd=off
  Reinterp1 : xbsIndex_r3/Reinterpret  force_arith_type=on  arith_type=Unsigned  force_bin_pt=on  bin_pt=0  force_valid=on
  Reinterp2 : xbsIndex_r3/Reinterpret  force_arith_type=on  arith_type=Unsigned  force_bin_pt=on  bin_pt=0  force_valid=on
  Out : Outport
  wires:
  Reinterp2/1 -> Concat/2
  In2/1 -> Reinterp2/1
  Reinterp1/1 -> Concat/1
  In1/1 -> Reinterp1/1
  Concat/1 -> Out/1

== system meat_1024pt_bee2_fpv3/vacc1/Uncram ==
  In : Inport  Port=1  LatchInput=off
  Reinterp1 : xbsIndex_r3/Reinterpret  force_arith_type=on  arith_type=Unsigned  force_bin_pt=on  bin_pt=31  force_valid=on
  Reinterp2 : xbsIndex_r3/Reinterpret  force_arith_type=on  arith_type=Unsigned  force_bin_pt=on  bin_pt=31  force_valid=on
  Slice1 : xbsIndex_r3/Slice  mode=Upper Bit Location + Width  nbits=32  bit1=0  base1=MSB of Input  bit0=0  base0=LSB of Input  boolean_output=off  explicit_period=off  period=1  dbl_ovrd=off
  Slice2 : xbsIndex_r3/Slice  mode=Upper Bit Location + Width  nbits=32  bit1=-32  base1=MSB of Input  bit0=0  base0=LSB of Input  boolean_output=off  explicit_period=off  period=1  dbl_ovrd=off
  Out1 : Outport
  Out2 : Outport  Port=2
  wires:
  In/1 -> Slice1/1, Slice2/1
  Slice1/1 -> Reinterp1/1
  Reinterp1/1 -> Out1/1
  Slice2/1 -> Reinterp2/1
  Reinterp2/1 -> Out2/1

== system meat_1024pt_bee2_fpv3/vacc1/vacc_core1 ==
  note: This BRAM and counter is exactly what is inside the green
      | Delay BRAM block. The functionality was extracted to avoid
      | library issues.
  din : Inport  Port=1  LatchInput=off
  acc_en : Inport  Port=2  LatchInput=off
  Adder : xbsIndex_r3/AddSub  mode=Addition  precision=User Defined  arith_type=Unsigned  n_bits=48  bin_pt=31  quantization=Truncate  overflow=Wrap  latency=2  explicit_period=on  period=1  use_carryin=off  use_carryout=off  en=off  dbl_ovrd=off  show_param=on  use_core=on  pipeline=on  use_rpm=on  gen_core=off
      settings: xl_area=[0, 0, 0, 0, 0, 0, 0]
  BRAM : xbsIndex_r3/Single Port RAM  depth=1024  initVector=0  write_mode=Read Before Write  latency=2  init_zero=on  explicit_period=off  period=1  rst=off  init_reg=0  en=off  dbl_ovrd=off  show_param=off  distributed_mem=off  use_rpm=off  gen_core=off
      settings: xl_area=[0, 0, 0, 0, 0, 0, 0]
  Constant : xbsIndex_r3/Constant  const=0  equ=P=C  arith_type=Unsigned  n_bits=1  bin_pt=0  opselect=C  inp2=PCIN>>17  opr=+  inp1=P  carry=CIN  iostate=0  explicit_period=off  period=1  dbl_ovrd=off
  Constant2 : xbsIndex_r3/Constant  const=1  equ=P=C  arith_type=Boolean  n_bits=1  bin_pt=0  opselect=C  inp2=PCIN>>17  opr=+  inp1=P  carry=CIN  iostate=0  explicit_period=on  period=1  dbl_ovrd=off
  Counter : xbsIndex_r3/Counter  cnt_type=Count Limited  n_bits=10  bin_pt=0  arith_type=Unsigned  start_count=0  cnt_to=1018  cnt_by_val=1  operation=Up  explicit_period=off  period=1  load_pin=off  rst=off  en=off  dbl_ovrd=off  show_param=off  use_rpm=off  gen_core=on
      settings: xl_area=[0, 0, 0, 0, 0, 0, 0]
  Mux : xbsIndex_r3/Mux  inputs=2  precision=Full  arith_type="Signed  (2's comp)"  n_bits=8  bin_pt=2  quantization=Truncate  overflow=Wrap  latency=1  explicit_period=off  period=1  en=off  dbl_ovrd=off  show_param=on  mux_type=off  use_rpm=on  gen_core=off
      settings: xl_area=[0, 0, 0, 0, 0, 0, 0]
  dout : Outport
  wires:
  Constant2/1 -> BRAM/3
  Counter/1 -> BRAM/1
  Adder/1 -> BRAM/2, dout/1
  Mux/1 -> Adder/2
  din/1 -> Adder/1
  BRAM/1 -> Mux/3
  Constant/1 -> Mux/2
  acc_en/1 -> Mux/1

== system meat_1024pt_bee2_fpv3/vacc1/vacc_core2 ==
  note: This BRAM and counter is exactly what is inside the green
      | Delay BRAM block. The functionality was extracted to avoid
      | library issues.
  din : Inport  Port=1  LatchInput=off
  acc_en : Inport  Port=2  LatchInput=off
  Adder : xbsIndex_r3/AddSub  mode=Addition  precision=User Defined  arith_type=Unsigned  n_bits=48  bin_pt=31  quantization=Truncate  overflow=Wrap  latency=2  explicit_period=on  period=1  use_carryin=off  use_carryout=off  en=off  dbl_ovrd=off  show_param=on  use_core=on  pipeline=on  use_rpm=on  gen_core=off
      settings: xl_area=[0, 0, 0, 0, 0, 0, 0]
  BRAM : xbsIndex_r3/Single Port RAM  depth=1024  initVector=0  write_mode=Read Before Write  latency=2  init_zero=on  explicit_period=off  period=1  rst=off  init_reg=0  en=off  dbl_ovrd=off  show_param=off  distributed_mem=off  use_rpm=off  gen_core=off
      settings: xl_area=[0, 0, 0, 0, 0, 0, 0]
  Constant : xbsIndex_r3/Constant  const=0  equ=P=C  arith_type=Unsigned  n_bits=1  bin_pt=0  opselect=C  inp2=PCIN>>17  opr=+  inp1=P  carry=CIN  iostate=0  explicit_period=off  period=1  dbl_ovrd=off
  Constant2 : xbsIndex_r3/Constant  const=1  equ=P=C  arith_type=Boolean  n_bits=1  bin_pt=0  opselect=C  inp2=PCIN>>17  opr=+  inp1=P  carry=CIN  iostate=0  explicit_period=on  period=1  dbl_ovrd=off
  Counter : xbsIndex_r3/Counter  cnt_type=Count Limited  n_bits=10  bin_pt=0  arith_type=Unsigned  start_count=0  cnt_to=1018  cnt_by_val=1  operation=Up  explicit_period=off  period=1  load_pin=off  rst=off  en=off  dbl_ovrd=off  show_param=off  use_rpm=off  gen_core=on
      settings: xl_area=[0, 0, 0, 0, 0, 0, 0]
  Mux : xbsIndex_r3/Mux  inputs=2  precision=Full  arith_type="Signed  (2's comp)"  n_bits=8  bin_pt=2  quantization=Truncate  overflow=Wrap  latency=1  explicit_period=off  period=1  en=off  dbl_ovrd=off  show_param=on  mux_type=off  use_rpm=on  gen_core=off
      settings: xl_area=[0, 0, 0, 0, 0, 0, 0]
  dout : Outport
  wires:
  Constant2/1 -> BRAM/3
  Counter/1 -> BRAM/1
  Adder/1 -> BRAM/2, dout/1
  Mux/1 -> Adder/2
  din/1 -> Adder/1
  BRAM/1 -> Mux/3
  Constant/1 -> Mux/2
  acc_en/1 -> Mux/1

== system meat_1024pt_bee2_fpv3/vacc2/Cram ==
  In1 : Inport  Port=1  LatchInput=off
  In2 : Inport  Port=2  LatchInput=off
  Concat : xbsIndex_r3/Concat  num_inputs=2  explicit_period=off  period=1  dbl_ovrd=off
  Reinterp1 : xbsIndex_r3/Reinterpret  force_arith_type=on  arith_type=Unsigned  force_bin_pt=on  bin_pt=0  force_valid=on
  Reinterp2 : xbsIndex_r3/Reinterpret  force_arith_type=on  arith_type=Unsigned  force_bin_pt=on  bin_pt=0  force_valid=on
  Out : Outport
  wires:
  Concat/1 -> Out/1
  In1/1 -> Reinterp1/1
  Reinterp1/1 -> Concat/1
  In2/1 -> Reinterp2/1
  Reinterp2/1 -> Concat/2

== system meat_1024pt_bee2_fpv3/vacc2/Uncram ==
  In : Inport  Port=1  LatchInput=off
  Reinterp1 : xbsIndex_r3/Reinterpret  force_arith_type=on  arith_type=Unsigned  force_bin_pt=on  bin_pt=46  force_valid=on
  Reinterp2 : xbsIndex_r3/Reinterpret  force_arith_type=on  arith_type=Unsigned  force_bin_pt=on  bin_pt=46  force_valid=on
  Slice1 : xbsIndex_r3/Slice  mode=Upper Bit Location + Width  nbits=48  bit1=0  base1=MSB of Input  bit0=0  base0=LSB of Input  boolean_output=off  explicit_period=off  period=1  dbl_ovrd=off
  Slice2 : xbsIndex_r3/Slice  mode=Upper Bit Location + Width  nbits=48  bit1=-48  base1=MSB of Input  bit0=0  base0=LSB of Input  boolean_output=off  explicit_period=off  period=1  dbl_ovrd=off
  Out1 : Outport
  Out2 : Outport  Port=2
  wires:
  In/1 -> Slice1/1, Slice2/1
  Slice1/1 -> Reinterp1/1
  Reinterp1/1 -> Out1/1
  Slice2/1 -> Reinterp2/1
  Reinterp2/1 -> Out2/1

== system meat_1024pt_bee2_fpv3/vacc2/vacc_core1 ==
  note: This BRAM and counter is exactly what is inside the green
      | Delay BRAM block. The functionality was extracted to avoid
      | library issues.
  din : Inport  Port=1  LatchInput=off
  acc_en : Inport  Port=2  LatchInput=off
  Adder : xbsIndex_r3/AddSub  mode=Addition  precision=User Defined  arith_type=Unsigned  n_bits=64  bin_pt=46  quantization=Truncate  overflow=Wrap  latency=2  explicit_period=on  period=1  use_carryin=off  use_carryout=off  en=off  dbl_ovrd=off  show_param=on  use_core=on  pipeline=on  use_rpm=on  gen_core=off
      settings: xl_area=[0, 0, 0, 0, 0, 0, 0]
  BRAM : xbsIndex_r3/Single Port RAM  depth=1024  initVector=0  write_mode=Read Before Write  latency=2  init_zero=on  explicit_period=off  period=1  rst=off  init_reg=0  en=off  dbl_ovrd=off  show_param=off  distributed_mem=off  use_rpm=off  gen_core=off
      settings: xl_area=[0, 0, 0, 0, 0, 0, 0]
  Constant : xbsIndex_r3/Constant  const=0  equ=P=C  arith_type=Unsigned  n_bits=1  bin_pt=0  opselect=C  inp2=PCIN>>17  opr=+  inp1=P  carry=CIN  iostate=0  explicit_period=off  period=1  dbl_ovrd=off
  Constant2 : xbsIndex_r3/Constant  const=1  equ=P=C  arith_type=Boolean  n_bits=1  bin_pt=0  opselect=C  inp2=PCIN>>17  opr=+  inp1=P  carry=CIN  iostate=0  explicit_period=on  period=1  dbl_ovrd=off
  Counter : xbsIndex_r3/Counter  cnt_type=Count Limited  n_bits=10  bin_pt=0  arith_type=Unsigned  start_count=0  cnt_to=1018  cnt_by_val=1  operation=Up  explicit_period=off  period=1  load_pin=off  rst=off  en=off  dbl_ovrd=off  show_param=off  use_rpm=off  gen_core=on
      settings: xl_area=[0, 0, 0, 0, 0, 0, 0]
  Mux : xbsIndex_r3/Mux  inputs=2  precision=Full  arith_type="Signed  (2's comp)"  n_bits=8  bin_pt=2  quantization=Truncate  overflow=Wrap  latency=1  explicit_period=off  period=1  en=off  dbl_ovrd=off  show_param=on  mux_type=off  use_rpm=on  gen_core=off
      settings: xl_area=[0, 0, 0, 0, 0, 0, 0]
  dout : Outport
  wires:
  acc_en/1 -> Mux/1
  Constant/1 -> Mux/2
  BRAM/1 -> Mux/3
  din/1 -> Adder/1
  Mux/1 -> Adder/2
  Adder/1 -> dout/1, BRAM/2
  Counter/1 -> BRAM/1
  Constant2/1 -> BRAM/3

== system meat_1024pt_bee2_fpv3/vacc2/vacc_core2 ==
  note: This BRAM and counter is exactly what is inside the green
      | Delay BRAM block. The functionality was extracted to avoid
      | library issues.
  din : Inport  Port=1  LatchInput=off
  acc_en : Inport  Port=2  LatchInput=off
  Adder : xbsIndex_r3/AddSub  mode=Addition  precision=User Defined  arith_type=Unsigned  n_bits=64  bin_pt=46  quantization=Truncate  overflow=Wrap  latency=2  explicit_period=on  period=1  use_carryin=off  use_carryout=off  en=off  dbl_ovrd=off  show_param=on  use_core=on  pipeline=on  use_rpm=on  gen_core=off
      settings: xl_area=[0, 0, 0, 0, 0, 0, 0]
  BRAM : xbsIndex_r3/Single Port RAM  depth=1024  initVector=0  write_mode=Read Before Write  latency=2  init_zero=on  explicit_period=off  period=1  rst=off  init_reg=0  en=off  dbl_ovrd=off  show_param=off  distributed_mem=off  use_rpm=off  gen_core=off
      settings: xl_area=[0, 0, 0, 0, 0, 0, 0]
  Constant : xbsIndex_r3/Constant  const=0  equ=P=C  arith_type=Unsigned  n_bits=1  bin_pt=0  opselect=C  inp2=PCIN>>17  opr=+  inp1=P  carry=CIN  iostate=0  explicit_period=off  period=1  dbl_ovrd=off
  Constant2 : xbsIndex_r3/Constant  const=1  equ=P=C  arith_type=Boolean  n_bits=1  bin_pt=0  opselect=C  inp2=PCIN>>17  opr=+  inp1=P  carry=CIN  iostate=0  explicit_period=on  period=1  dbl_ovrd=off
  Counter : xbsIndex_r3/Counter  cnt_type=Count Limited  n_bits=10  bin_pt=0  arith_type=Unsigned  start_count=0  cnt_to=1018  cnt_by_val=1  operation=Up  explicit_period=off  period=1  load_pin=off  rst=off  en=off  dbl_ovrd=off  show_param=off  use_rpm=off  gen_core=on
      settings: xl_area=[0, 0, 0, 0, 0, 0, 0]
  Mux : xbsIndex_r3/Mux  inputs=2  precision=Full  arith_type="Signed  (2's comp)"  n_bits=8  bin_pt=2  quantization=Truncate  overflow=Wrap  latency=1  explicit_period=off  period=1  en=off  dbl_ovrd=off  show_param=on  mux_type=off  use_rpm=on  gen_core=off
      settings: xl_area=[0, 0, 0, 0, 0, 0, 0]
  dout : Outport
  wires:
  acc_en/1 -> Mux/1
  Constant/1 -> Mux/2
  BRAM/1 -> Mux/3
  din/1 -> Adder/1
  Mux/1 -> Adder/2
  Adder/1 -> dout/1, BRAM/2
  Counter/1 -> BRAM/1
  Constant2/1 -> BRAM/3
